simulink model "Pitch_on_Roll__Sim"  (R2024b)
settings: Solver=VariableStepAuto  StartTime=0.0  StopTime=sysParams.Simulation.tSim  RelTol=1e-3  AbsTol=1e-3  EnableMultiTasking=on
undefined symbols (not defined in the file or in its folder): baseAccEcho, baseRatesEcho, gyro, innerAxisMetry, MassProps, outerAxisMetry, X, Y, Z
libraries: sm_lib x11, nesl_utility x8, Pitch_on_Roll__Lib x4, fl_lib x2, matrix_library x2
settings Model: Creator=leoni  LastModifiedBy=leoni
settings SolverCC: AutoScaleAbsTol=off  AlgebraicLoopSolver=TrustRegion  MaxZcPerStep=1
settings DataIOCC: LimitDataPoints=on  MaxDataPoints=10000
settings OptimizationCC: ReuseModelBlockBuffer=off  LifeSpan=inf
settings DebuggingCC: UnconnectedInputMsg=warning  UnconnectedOutputMsg=warning  UnconnectedLineMsg=warning  AllowSymbolicDim=off  SubsystemReferenceDiagnosticForUnitTest=warning  SFUnexpectedBacktrackingDiag=warning  SFNoUnconditionalDefaultTransitionDiag=warning  SFExecutionAtInitializationDiag=none  ArithmeticOperatorsInVariantConditions=warning
settings ModelReferenceCC: EnableRefExpFcnMdlSchedulingChecks=on
settings SFSimCC: SimUseLocalCustomCode=off  CustomCodeUndefinedFunction=UseInterfaceOnly
settings RTWCC: RTWUseLocalCustomCode=off  GPUComputeCapability=3.5  DLArmComputeVersion=19.05
settings CodeAppCC: StateflowObjectComments=on
settings GRTTargetCC: TargetLangStandard=C89/C90 (ANSI)
settings ConfigComp: CovMetricSettings=dw  CovSaveCumulativeToWorkspaceVar=on  CovSaveSingleToWorkspaceVar=on  CovExternalEMLEnable=off  CovSFcnEnable=off
settings SimscapeCC: SimscapeLogType=all  SimscapeLogSimulationStatistics=on  SimscapeLogDataHistory=10000

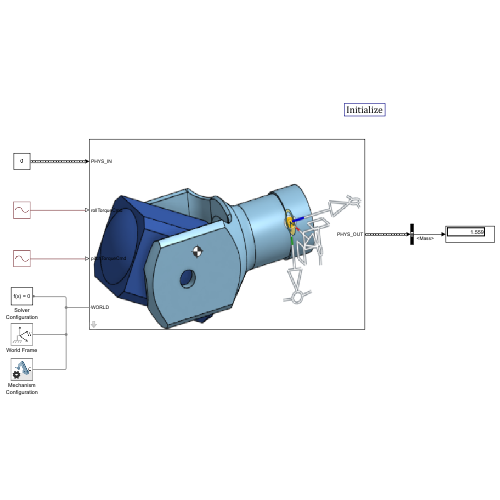
[thumbnail: Simulink's stored preview of the top-level diagram]
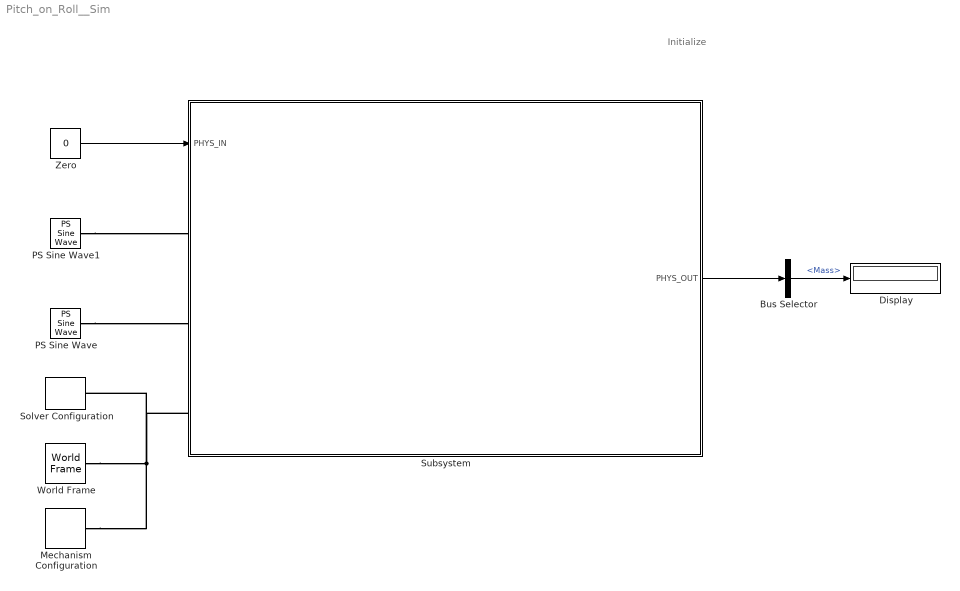
== system Pitch_on_Roll__Sim ==
  note: Initialize
  Bus Selector : BusSelector  OutputSignals=outerAxisMetry.MassProps.Mass
  Display : Display
  Mechanism Configuration : sm_lib/Utilities/Mechanism Configuration  UniformGravity=None  GravityVector=[0 0 -9.80665]  GravityVectorUnits=m/s^2  LinearizationDelta=0.001  JointModeTransitionNonlinearIterations=2
  PS Sine Wave : fl_lib/Physical Signals/Sources/PS Sine Wave  amplitude=20 N*mm  bias=0  frequency_spec=foundation.enum.frequencySpec.frequencySI  frequency_SI=1 Hz  frequency_angular=1 rad/s  phase=0 rad
      settings: InternalSimscapePortConfiguration="{\"Bottom\":[],\"Left\":[],\"Right\":[{\"id\":\"O\",\"label\":\"\",\"type\":\"output\"}],\"Top\":[]}"
  PS Sine Wave1 : fl_lib/Physical Signals/Sources/PS Sine Wave  amplitude=100 N*mm  bias=0  frequency_spec=foundation.enum.frequencySpec.frequencySI  frequency_SI=2 Hz  frequency_angular=1 rad/s  phase=0 rad
      settings: InternalSimscapePortConfiguration="{\"Bottom\":[],\"Left\":[],\"Right\":[{\"id\":\"O\",\"label\":\"\",\"type\":\"output\"}],\"Top\":[]}"
  Solver Configuration : nesl_utility/Solver Configuration  PhysicalDomain=network_engine_domain  SubClassName=solver  LeftPortType=input  RightPortType=generic  Tones=[]  Harmonics=[]  SimulateNoise=off  Profile=off  UseLocalSampling=off  EnableSwitchedLinearOptims=on  FrequencyDomain=off  UseCCode=off  RelTol=0.001  AbsTol=1e-06  MinStep=1e-09  ToWorkspace=off  RevertToSquareIcSolve=off  NumHomotopyIterations=100  PhasorMode=off  PhasorModeNumHarmonics=1  ConsistencySolver=NEWTON_XTOL_AFTER_FTOL  IndexReductionMethod=DerivativeReplacement  DoDC=off  ResidualTolerance=1e-09  ConsistencyTolSource=GLOBAL  ConsistencyAbsTol=0.001  ConsistencyRelTol=0.001  ConsistencyTolFactor=0.001  UseLocalSolver=off  LocalSolverChoice=NE_TRAPEZOIDAL_ADVANCER  ResolveIndetEquations=on  FunctionEvalNumThread=1  LocalSolverSampleTime=0.001  DoFixedCost=off  MaxNonlinIter=3  MaxModeIter=2  ComputeImpulses=off  ImpulseIterations=2  LinearAlgebra=Sparse  LinearAlgebraNumThread=0  EquationFormulation=NE_TIME_EF  DelaysMemoryBudget=1024  AutomaticFiltering=on  FilteringTimeConstant=0.001  PartitionStorageMethod=AS_NEEDED  PartitionMemoryBudget=1024  PartitionMethod=FAST  MultibodyUseLocalSolver=off  MultibodyLocalSolverChoice=ODE2  MultibodyLocalSolverSampleTime=0.001
  Subsystem : Subsystem  mask{isRigidModel=on, nModes=10}
      mask prompts: isRigidModel "Rigid Meachanics Active"; nModes "Number of Modes"
      mask DialogControl Container3 Prompt: Gimbals Modeling Properties
      mask Display: image('Pitch_on_Roll__image.png');
  World Frame : sm_lib/Frames and Transforms/World Frame
  Zero : Constant  Value=0  OutDataTypeStr=Bus: PHYS_IN
  wires:
  Zero/1 -> Subsystem/1(PHYS_IN)
  Subsystem/1(PHYS_OUT) -> Bus Selector/1
  Bus Selector/1 -> Display/1  "<Mass>"
  connections:
  Mechanism Configuration/RConn1 -- Subsystem/LConn3 -- Solver Configuration/RConn1 -- World Frame/RConn1
  PS Sine Wave/RConn1 -- Subsystem/LConn2
  PS Sine Wave1/RConn1 -- Subsystem/LConn1

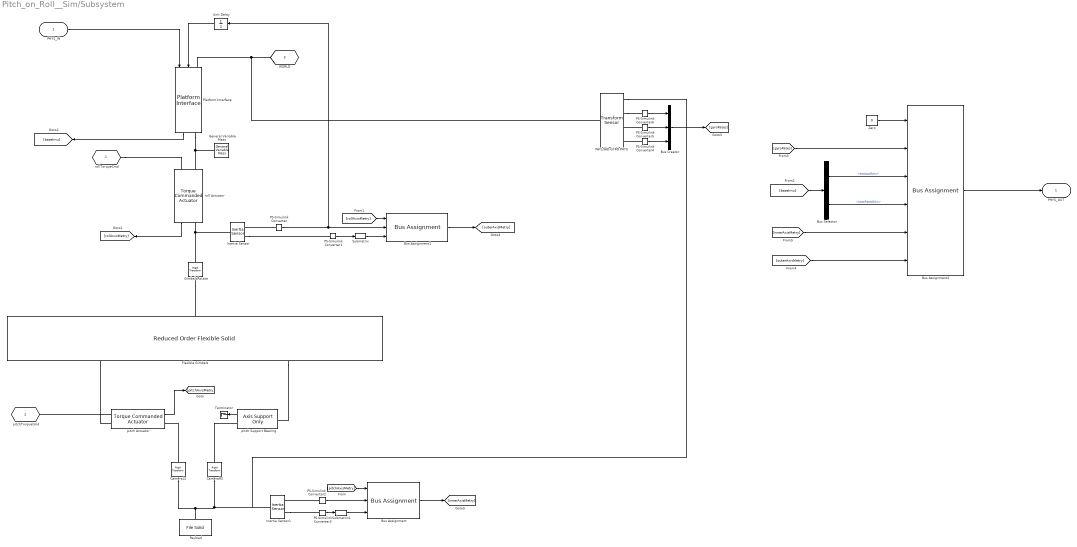
== system Pitch_on_Roll__Sim/Subsystem ==
  PHYS_IN : Inport  OutDataTypeStr=Bus: PHYS_IN
  Bus Assignment : BusAssignment  AssignedSignals=MassProps.Mass,MassProps.Inertia
  Bus Assignment1 : BusAssignment  AssignedSignals=MassProps.Mass,MassProps.Inertia
  Bus Assignment2 : BusAssignment  AssignedSignals=gyro,baseAccEcho,baseRatesEcho,innerAxisMetry,outerAxisMetry
  Bus Creator : BusCreator  Inputs=3  OutDataTypeStr=Bus: rates
      settings: InheritFromInputs=off
  Bus Selector : BusSelector  OutputSignals=baseAccEcho,baseRatesEcho
  CameraLS : sm_lib/Frames and Transforms/Rigid Transform  RotationMethod=AlignedAxes  FollAlignAxisA=+Z  BaseAlignAxisA=+Z  FollAlignAxisB=+Y  BaseAlignAxisB=+X  RotationStandardAxis=+Z  RotationAngle=0  RotationAngleUnits=deg  RotationArbitraryAxis=[0 0 1]  RotationSequenceAxes=FollowerAxes  RotationSequence=XYX  RotationSequenceAngles=[0 0 0]  RotationSequenceAnglesUnits=deg  RotationMatrix=[1 0 0;0 1 0;0 0 1]  Quaternion=[1 0 0 0]  TranslationMethod=Cartesian  TranslationCartesianOffset=[0 0 -25]  TranslationCartesianOffsetUnits=mm  TranslationStandardAxis=+Z  TranslationStandardOffset=0  TranslationStandardOffsetUnits=m  TranslationROffset=0  TranslationROffsetUnits=m  TranslationThetaOffset=0  TranslationThetaOffsetUnits=deg  TranslationZOffset=0  TranslationZOffsetUnits=m
  CameraRS : sm_lib/Frames and Transforms/Rigid Transform  RotationMethod=AlignedAxes  FollAlignAxisA=+Z  BaseAlignAxisA=+Z  FollAlignAxisB=+Y  BaseAlignAxisB=+X  RotationStandardAxis=+Z  RotationAngle=0  RotationAngleUnits=deg  RotationArbitraryAxis=[0 0 1]  RotationSequenceAxes=FollowerAxes  RotationSequence=XYX  RotationSequenceAngles=[0 0 0]  RotationSequenceAnglesUnits=deg  RotationMatrix=[1 0 0;0 1 0;0 0 1]  Quaternion=[1 0 0 0]  TranslationMethod=Cartesian  TranslationCartesianOffset=[0 0 25]  TranslationCartesianOffsetUnits=mm  TranslationStandardAxis=+Z  TranslationStandardOffset=0  TranslationStandardOffsetUnits=m  TranslationROffset=0  TranslationROffsetUnits=m  TranslationThetaOffset=0  TranslationThetaOffsetUnits=deg  TranslationZOffset=0  TranslationZOffsetUnits=m
  Flexible Gimbals : sm_lib/Body Elements/Flexible Bodies/Reduced Order Flexible Solid  UnitSystemType=Custom  LengthUnit=mm  MassUnit=kg  TimeUnit=s  NumberOfInterfaceFrames=3  InterfaceFrameOrigins=gimbals.P  InterfaceFrameOrientations=[1 0 0 0;1 0 0 0;1 0 0 0]  StiffnessMatrix=gimbals.K  MassMatrix=gimbals.M  DampingType=DampingMatrix  ProportionalDampingAlpha=0  ProportionalDampingBeta=0.001  UniformModalDampingRatio=0.01  DampingMatrix=gimbals.C  ReductionType=ModallyReduced  NumRetainedModes=nModes*(~isRigidModel)  GraphicType=PartitionedGeometry  GeomFileName=D:\Git\Pitch_on_Roll\Models\GImbals.step  GeomUnitType=FromFile  VisRecursionLimit=3  GraphicVertexCoordinates=[]  GraphicFacetVertexIndices=[]  GraphicReconstructionMatrix=[]  GraphicVisPropType=FromFileVisualProperties  GraphicDiffuseColor=[0.5 0.5 0.5]  GraphicOpacity=1  GraphicSpecularColor=[0.5 0.5 0.5 1.0]  GraphicAmbientColor=[0.15 0.15 0.15 1.0]  GraphicEmissiveColor=[0.0 0.0 0.0 1.0]  GraphicShininess=75
  General Variable Mass : sm_lib/Body Elements/Variable Mass/General Variable Mass  VariableInertiaType=Custom  MassType=Constant  Mass=1  MassUnits=g  CenterOfMassType=Constant  CenterOfMass=[0 0 0]  CenterOfMassUnits=m  InertiaMatrixType=Constant  MomentsOfInertia=[1 1 1]  MomentsOfInertiaUnits=kg*m^2  ProductsOfInertia=[0 0 0]  ProductsOfInertiaUnits=kg*m^2  GraphicType=Marker  MarkerShape=Sphere  MarkerSize=10  GraphicVisPropType=SimpleVisualProperties  GraphicDiffuseColor=[0.5 0.5 0.5]  GraphicOpacity=1  GraphicSpecularColor=[0.5 0.5 0.5 1.0]  GraphicAmbientColor=[0.15 0.15 0.15 1.0]  GraphicEmissiveColor=[0.0 0.0 0.0 1.0]  GraphicShininess=75
  GimbalsRotate : sm_lib/Frames and Transforms/Rigid Transform  RotationMethod=AlignedAxes  FollAlignAxisA=+X  BaseAlignAxisA=+Z  FollAlignAxisB=+Y  BaseAlignAxisB=+Y  RotationStandardAxis=+Z  RotationAngle=0  RotationAngleUnits=deg  RotationArbitraryAxis=[0 0 1]  RotationSequenceAxes=FollowerAxes  RotationSequence=XYX  RotationSequenceAngles=[0 0 0]  RotationSequenceAnglesUnits=deg  RotationMatrix=[1 0 0;0 1 0;0 0 1]  Quaternion=[1 0 0 0]  TranslationMethod=None  TranslationCartesianOffset=[0 0 -25]  TranslationCartesianOffsetUnits=mm  TranslationStandardAxis=+Z  TranslationStandardOffset=0  TranslationStandardOffsetUnits=m  TranslationROffset=0  TranslationROffsetUnits=m  TranslationThetaOffset=0  TranslationThetaOffsetUnits=deg  TranslationZOffset=0  TranslationZOffsetUnits=m
  Inertia Sensor : sm_lib/Body Elements/Inertia Sensor  SensorExtent=Mechanism  SpanWeldJoints=off  ExcludeGroundedBodies=off  MeasurementFrame=Attached  SenseMass=on  SenseCenterOfMass=off  SenseInertiaMatrix=on  SenseCenteredInertiaMatrix=off  SensePrincipalInertiaMatrix=off  SenseRotationMatrix=off  GraphicType=PrincipalInertiaFrame  PrincipalInertiaFrameSize=20  GraphicVisPropType=AdvancedVisualProperties  GraphicDiffuseColor=[0.5 0.5 0.5]  GraphicOpacity=1  GraphicSpecularColor=[0.5 0.5 0.5 1.0]  GraphicAmbientColor=[0.15 0.15 0.15 1.0]  GraphicEmissiveColor=[0.0 0.0 0.0 1.0]  GraphicShininess=75
  Inertia Sensor1 : sm_lib/Body Elements/Inertia Sensor  SensorExtent=BodyGroup  SpanWeldJoints=off  ExcludeGroundedBodies=on  MeasurementFrame=Attached  SenseMass=on  SenseCenterOfMass=off  SenseInertiaMatrix=on  SenseCenteredInertiaMatrix=off  SensePrincipalInertiaMatrix=off  SenseRotationMatrix=off  GraphicType=PrincipalInertiaFrame  PrincipalInertiaFrameSize=20  GraphicVisPropType=AdvancedVisualProperties  GraphicDiffuseColor=[0.5 0.5 0.5]  GraphicOpacity=1  GraphicSpecularColor=[0.5 0.5 0.5 1.0]  GraphicAmbientColor=[0.15 0.15 0.15 1.0]  GraphicEmissiveColor=[0.0 0.0 0.0 1.0]  GraphicShininess=75
  PAYLOAD GYRO PHYS : sm_lib/Frames and Transforms/Transform Sensor  MeasurementFrame=World  RotationSequence=YXZ  SenseAngle=off  SenseAxis=off  SenseQ=off  SenseR=off  SenseRotationSequence=off  SenseOmegaX=on  SenseOmegaY=on  SenseOmegaZ=on  SenseOmega=off  SenseQDot=off  SenseRDot=off  SenseRotationSequenceDot=off  SenseAlphaX=off  SenseAlphaY=off  SenseAlphaZ=off  SenseAlpha=off  SenseQDDot=off  SenseRDDot=off  SenseX=off  SenseY=off  SenseZ=off  SenseXYZ=off  SenseRad=off  SenseAzim=off  SenseDist=off  SenseInc=off  SenseXDot=off  SenseYDot=off  SenseZDot=off  SenseXYZDot=off  SenseRadDot=off  SenseAzimDot=off  SenseDistDot=off  SenseIncDot=off  SenseXDDot=off  SenseYDDot=off  SenseZDDot=off  SenseXYZDDot=off  SenseRadDDot=off  SenseAzimDDot=off  SenseDistDDot=off  SenseIncDDot=off
  PS-Simulink Converter : nesl_utility/PS-Simulink Converter  PhysicalDomain=network_engine_domain  SubClassName=ps_output  LeftPortType=input  RightPortType=output  PseudoPeriodic=off  Frequencies=[]  VectorFormat=inherit  Unit=kg  AffineConversion=off
  PS-Simulink Converter1 : nesl_utility/PS-Simulink Converter  PhysicalDomain=network_engine_domain  SubClassName=ps_output  LeftPortType=input  RightPortType=output  PseudoPeriodic=off  Frequencies=[]  VectorFormat=inherit  Unit=kg*mm^2  AffineConversion=off
  PS-Simulink Converter2 : nesl_utility/PS-Simulink Converter  PhysicalDomain=network_engine_domain  SubClassName=ps_output  LeftPortType=input  RightPortType=output  PseudoPeriodic=off  Frequencies=[]  VectorFormat=inherit  Unit=kg  AffineConversion=off
  PS-Simulink Converter3 : nesl_utility/PS-Simulink Converter  PhysicalDomain=network_engine_domain  SubClassName=ps_output  LeftPortType=input  RightPortType=output  PseudoPeriodic=off  Frequencies=[]  VectorFormat=inherit  Unit=kg*m^2  AffineConversion=off
  PS-Simulink Converter4 : nesl_utility/PS-Simulink Converter  PhysicalDomain=network_engine_domain  SubClassName=ps_output  LeftPortType=input  RightPortType=output  PseudoPeriodic=off  Frequencies=[]  VectorFormat=inherit  Unit=rad/s  AffineConversion=off
  PS-Simulink Converter5 : nesl_utility/PS-Simulink Converter  PhysicalDomain=network_engine_domain  SubClassName=ps_output  LeftPortType=input  RightPortType=output  PseudoPeriodic=off  Frequencies=[]  VectorFormat=inherit  Unit=rad/s  AffineConversion=off
  PS-Simulink Converter6 : nesl_utility/PS-Simulink Converter  PhysicalDomain=network_engine_domain  SubClassName=ps_output  LeftPortType=input  RightPortType=output  PseudoPeriodic=off  Frequencies=[]  VectorFormat=inherit  Unit=rad/s  AffineConversion=off
  Payload : sm_lib/Body Elements/File Solid  ExtGeomFileName=D:\Git\Pitch_on_Roll\Models\Camera.step  UnitType=FromFile  ExtGeomFileUnits=m  StepReaderType=HEX  ExportConvexHullGeometry=off  InertiaType=Custom  BasedOnType=DensityFromFile  Density=1000  DensityUnits=kg/m^3  Mass=1200  MassUnits=g  CenterOfMass=[0 0 0]  CenterOfMassUnits=mm  MomentsOfInertia=[1400 2500 2500]  MomentsOfInertiaUnits=kg*mm^2  ProductsOfInertia=[0 0 0]  ProductsOfInertiaUnits=kg*m^2  GraphicType=FromGeometry  MarkerShape=Sphere  MarkerSize=10  GraphicVisPropType=FromFileVisualProperties  GraphicDiffuseColor=[0.5 0.5 0.5]  GraphicOpacity=1  GraphicSpecularColor=[0.5 0.5 0.5 1.0]  GraphicAmbientColor=[0.15 0.15 0.15 1.0]  GraphicEmissiveColor=[0.0 0.0 0.0 1.0]  GraphicShininess=75  DoExposeReferenceFrame=on  SerializedFrames=<Frames/>
  Platform Interface : Pitch_on_Roll__Lib/Platform Interface  mappingX=X  mappingY=X  mappingZ=X  noBaseMotion=on
  Submatrix : matrix_library/Submatrix  RowSpan=One row  RowStartMode=Last  RowStartIndex=1  RowEndMode=Last  RowEndIndex=1  ColSpan=One column  ColStartMode=Last  ColStartIndex=1  ColEndMode=Last  ColEndIndex=1
  Submatrix1 : matrix_library/Submatrix  RowSpan=One row  RowStartMode=Last  RowStartIndex=1  RowEndMode=Last  RowEndIndex=1  ColSpan=One column  ColStartMode=Last  ColStartIndex=1  ColEndMode=Last  ColEndIndex=1
  Terminator : Terminator
  Unit Delay : UnitDelay  SampleTime=-1  HasFrameUpgradeWarning=on
  Zero : Constant  Value=0  OutDataTypeStr=Bus: PHYS_OUT
  pitch Actuator : Pitch_on_Roll__Lib/Torque Commanded Actuator  bearingProps=plantParams.pitchBearing  harnessConstant=plantParams.pitchHarnessSpring  noDist=on
  pitch Support Bearing : Pitch_on_Roll__Lib/Axis Support Only  bearingProps=plantParams.pitchBearing  noDist=on
  roll Actuator : Pitch_on_Roll__Lib/Torque Commanded Actuator  bearingProps=plantParams.rollBearing  harnessConstant=plantParams.rollHarnessSpring  noDist=on
  rollTorqueCmd : PMIOPort  Side=Left
  pitchTorqueCmd : PMIOPort  Port=2  Side=Left
  WORLD : PMIOPort  Port=3  Side=Left
  PHYS_OUT : Outport  OutDataTypeStr=Bus: PHYS_OUT
  wires:
  roll Actuator/1 -> [rollAxisMetry]
  pitch Actuator/1 -> [pitchAxisMetry]
  pitch Support Bearing/1 -> Terminator/1
  PS-Simulink Converter2/1 -> Bus Assignment/2
  PS-Simulink Converter3/1 -> Submatrix1/1
  Submatrix1/1 -> Bus Assignment/3
  [pitchAxisMetry] -> Bus Assignment/1
  Bus Assignment/1 -> [innerAxisMetry]
  PS-Simulink Converter/1 -> Unit Delay/1, Bus Assignment1/2
  PS-Simulink Converter1/1 -> Submatrix/1
  [rollAxisMetry] -> Bus Assignment1/1
  Submatrix/1 -> Bus Assignment1/3
  Bus Assignment1/1 -> [outerAxisMetry]
  Unit Delay/1 -> Platform Interface/2
  PHYS_IN/1 -> Platform Interface/1
  Platform Interface/1 -> [baseImu]
  PS-Simulink Converter5/1 -> Bus Creator/2
  PS-Simulink Converter4/1 -> Bus Creator/3
  PS-Simulink Converter6/1 -> Bus Creator/1
  Bus Creator/1 -> [gyroRates]
  Zero/1 -> Bus Assignment2/1
  [gyroRates] -> Bus Assignment2/2
  [baseImu] -> Bus Selector/1
  Bus Selector/2 -> Bus Assignment2/4  "<baseRatesEcho>"
  Bus Selector/1 -> Bus Assignment2/3  "<baseAccEcho>"
  [outerAxisMetry] -> Bus Assignment2/6
  [innerAxisMetry] -> Bus Assignment2/5
  Bus Assignment2/1 -> PHYS_OUT/1
  connections:
  CameraRS/LConn1 -- pitch Support Bearing/RConn1
  Inertia Sensor/LConn1 -- GimbalsRotate/LConn1 -- roll Actuator/RConn1
  pitch Actuator/LConn2 -- Flexible Gimbals/LConn1
  CameraLS/RConn1 -- PAYLOAD GYRO PHYS/RConn1 -- Inertia Sensor1/LConn1 -- CameraRS/RConn1 -- Payload/RConn1
  CameraLS/LConn1 -- pitch Actuator/RConn1
  rollTorqueCmd/RConn1 -- roll Actuator/LConn1
  pitch Actuator/LConn1 -- pitchTorqueCmd/RConn1
  PS-Simulink Converter2/LConn1 -- Inertia Sensor1/RConn1
  Inertia Sensor1/RConn2 -- PS-Simulink Converter3/LConn1
  PS-Simulink Converter/LConn1 -- Inertia Sensor/RConn1
  Inertia Sensor/RConn2 -- PS-Simulink Converter1/LConn1
  Flexible Gimbals/LConn2 -- pitch Support Bearing/LConn1
  Flexible Gimbals/RConn1 -- GimbalsRotate/RConn1
  WORLD/RConn1 -- PAYLOAD GYRO PHYS/LConn1 -- Platform Interface/LConn1
  PS-Simulink Converter4/LConn1 -- PAYLOAD GYRO PHYS/RConn4
  PS-Simulink Converter5/LConn1 -- PAYLOAD GYRO PHYS/RConn3
  PAYLOAD GYRO PHYS/RConn2 -- PS-Simulink Converter6/LConn1
  Platform Interface/RConn1 -- General Variable Mass/RConn1 -- roll Actuator/LConn2
